simulink model "EulerPIDTunning"  (Simulink 7.6)
settings: Solver=ode3  StartTime=0.0  StopTime=2  FixedStep=Ts  RelTol=1e-3
InitFcn:
  | eval('Config');
  | eval('RobotCtlCfg');
values from neighbouring files (symbols this model uses):
  a2 = 0    [Config.m]    (also in CtrPlatformCfg.m)
  a3 = 0    [Config.m]    (also in CtrPlatformCfg.m)
  a4 = 0    [Config.m]    (also in CtrPlatformCfg.m)
  a5 = 90    [Config.m]    (also in CtrPlatformCfg.m)
  a6 = 0    [Config.m]    (also in CtrPlatformCfg.m)
  freq = tvel/radius    (= 1)    [Config.m]    (also in CtrPlatformCfg.m)
  Gravity = 9.8    [Config.m]    (also in CtrPlatformCfg.m)
  in1 = [5.2954 -0.2565 -0.6366;-0.2565 4.7000 0.2830;-0.6366 0.2829 5.8635]    [Config.m]    (also in CtrPlatformCfg.m; DynEulerTest.m; EfDynCAD.m = [0.54  -0.01 0.23)
  in2 = [5.8840 0.0072 0.0135;0.0072 6.0178 -0.1907;0.0135 -0.1907 0.3374]    [Config.m]    (also in CtrPlatformCfg.m; DynEulerTest.m; EfDynCAD.m = (R_x*R_z)*in2*(R_x*R_z)')
  in3 = [1.8201 -0.2274 -0.3112;-0.2274 2.2537 -0.1441;-0.3112 -0.1441 1.9485]    [Config.m]    (also in CtrPlatformCfg.m; DynEulerTest.m; EfDynCAD.m = (R_x*R_z)*in3*(R_x*R_z)')
  in4 = [0.0607 -0.0922 0;-0.0922 1.4493 0;0 0 1.4620]    [Config.m]    (also in CtrPlatformCfg.m; DynEulerTest.m = [0.0607 -0.0922 0;-0.0922 1.4493 0;0 0,1.4620]; EfDynCAD.m = (R_y*Rz)*in4*(R_y*Rz)')
  in5 = [0.0191 0.0032 0;0.0032 0.0228 0;0 0 0.0291]    [Config.m]    (also in CtrPlatformCfg.m; DynEulerTest.m; EfDynCAD.m = (R_x*R_y)*in5*(R_x*R_y)')
  in6 = [0.0012 0 0;0 0.0007 0;0 0 0.0007]    [Config.m]    (also in CtrPlatformCfg.m; DynEulerTest.m; EfDynCAD.m = (R_y*Rz)*in6*(R_y*Rz)')
  init_Endx = gd_init(1,4)    [Config.m]    (also in CtrPlatformCfg.m)
  init_Endy = gd_init(2,4)    [Config.m]    (also in CtrPlatformCfg.m)
  init_Endz = gd_init(3,4)    [Config.m]    (also in CtrPlatformCfg.m)
  init_Rot = gd_init(1:3,1:3)    [Config.m]    (also in CtrPlatformCfg.m)
  L = [l1 l2 l3 l4 l5 l6 l7 l8 l9]    [Config.m]    (also in CtrPlatformCfg.m)
  ma1 = 170.31    [Config.m]    (also in CtrPlatformCfg.m; DynEulerTest.m; EfDynCAD.m = 77.75)
  ma2 = 63.74    [Config.m]    (also in CtrPlatformCfg.m; DynEulerTest.m; EfDynCAD.m = 32.31)
  ma3 = 98.98    [Config.m]    (also in CtrPlatformCfg.m; DynEulerTest.m; EfDynCAD.m = 18.61)
  ma4 = 24.46    [Config.m]    (also in CtrPlatformCfg.m; DynEulerTest.m; EfDynCAD.m = 15.65)
  ma5 = 5.24    [Config.m]    (also in CtrPlatformCfg.m; DynEulerTest.m; EfDynCAD.m = 3.32)
  ma6 = 0.6    [Config.m]    (also in CtrPlatformCfg.m; DynEulerTest.m; EfDynCAD.m)
  Rad2Line = Gear*EncRes/(2*pi)    [Config.m]    (also in CtrPlatformCfg.m)
  Ts = 1/FrHz    (= 0.00025)    [Config.m]    (also in CtrPlatformCfg.m)
  tvel = 120    [Config.m]    (also in CtrPlatformCfg.m)
undefined symbols (not defined in the file or in its folder): a1, DiscIntNeverNeededParam, PRBSGain, PRBSOffset, PRBSTimeLength, PulseFrq, PulseGain, RobotAxis, SineFrq, SineGain, V2T
libraries: simulink x55, mblibv1 x35, powerlib_extras x7
(part 1 of 3)
settings Model: Creator=DAI Dan  LastModifiedBy=DAI Dan
settings SimMechanicsCC: VisOnUpdateDiagram=on

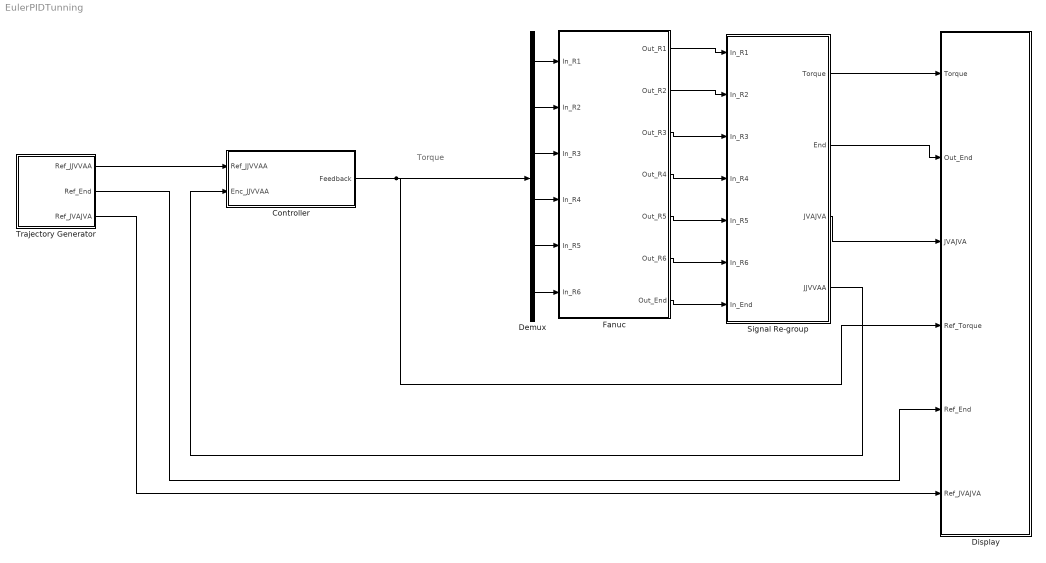
== system EulerPIDTunning ==
  note: Torque
  Controller : Subsystem
  Demux : Demux  Outputs=6
  Display : Subsystem
  Fanuc : Subsystem
  Signal Re-group : Subsystem
  Trajectory Generator : Subsystem
  wires:
  Fanuc/1(Out_R1) -> Signal Re-group/1(In_R1)
  Fanuc/2(Out_R2) -> Signal Re-group/2(In_R2)
  Fanuc/3(Out_R3) -> Signal Re-group/3(In_R3)
  Fanuc/4(Out_R4) -> Signal Re-group/4(In_R4)
  Fanuc/5(Out_R5) -> Signal Re-group/5(In_R5)
  Fanuc/6(Out_R6) -> Signal Re-group/6(In_R6)
  Fanuc/7(Out_End) -> Signal Re-group/7(In_End)
  Signal Re-group/4(JJVVAA) -> Controller/2(Enc_JJVVAA)
  Demux/1 -> Fanuc/1(In_R1)
  Demux/2 -> Fanuc/2(In_R2)
  Demux/3 -> Fanuc/3(In_R3)
  Demux/4 -> Fanuc/4(In_R4)
  Demux/5 -> Fanuc/5(In_R5)
  Demux/6 -> Fanuc/6(In_R6)
  Signal Re-group/1(Torque) -> Display/1(Torque)
  Signal Re-group/2(End) -> Display/2(Out_End)
  Signal Re-group/3(JVAJVA) -> Display/3(JVAJVA)
  Trajectory Generator/1(Ref_JJVVAA) -> Controller/1(Ref_JJVVAA)
  Trajectory Generator/2(Ref_End) -> Display/5(Ref_End)
  Trajectory Generator/3(Ref_JVAJVA) -> Display/6(Ref_JVAJVA)
  Controller/1(Feedback) -> Display/4(Ref_Torque), Demux/1

== system EulerPIDTunning/Controller ==
  note: Note:
      | AugPD controller
      |  Input: rad
      | Output: N*m
      | PID Controller
      | Input: rad-->lines
      | Output: N*m-->Current/Volt
  Ref_JJVVAA : Inport
  Enc_JJVVAA : Inport  Port=2
  PID Controller : Subsystem
  Terminator : Terminator
  Feedback : Outport
  wires:
  Ref_JJVVAA/1 -> PID Controller/1(Ref)
  Enc_JJVVAA/1 -> PID Controller/2(Enc)
  PID Controller/1(Feedback) -> Feedback/1
  PID Controller/2(ErrorFlag) -> Terminator/1

== system EulerPIDTunning/Display ==
  Torque : Inport
  Out_End : Inport  Port=2
  JVAJVA : Inport  Port=3
  Ref_Torque : Inport  Port=4
  Ref_End : Inport  Port=5
  Ref_JVAJVA : Inport  Port=6
  EndTrjDisplay : Subsystem
  JntVelAccDisplay : Subsystem
  TorqueDisplay : Subsystem
  wires:
  Torque/1 -> TorqueDisplay/1(Torque)
  Ref_Torque/1 -> TorqueDisplay/2(Ref_Torque)
  JVAJVA/1 -> JntVelAccDisplay/1(JointVelAcc)
  Ref_JVAJVA/1 -> JntVelAccDisplay/2(Ref_JntVelAcc)
  Out_End/1 -> EndTrjDisplay/1(End)
  Ref_End/1 -> EndTrjDisplay/2(RefEnd)

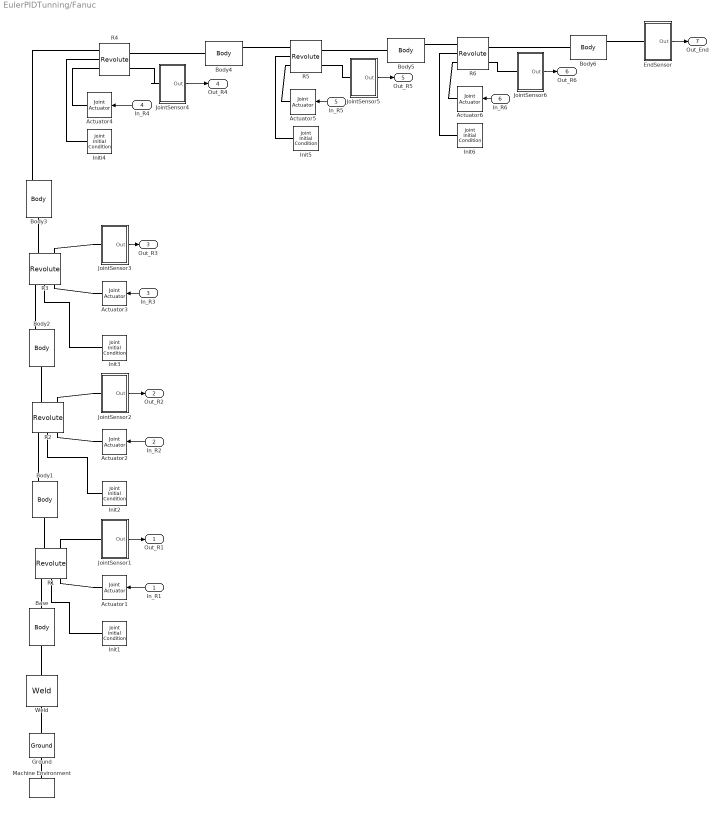
== system EulerPIDTunning/Fanuc ==
  In_R1 : Inport
  In_R2 : Inport  Port=2
  In_R3 : Inport  Port=3
  In_R4 : Inport  Port=4
  In_R5 : Inport  Port=5
  In_R6 : Inport  Port=6
  " EndSensor" : Subsystem
  Actuator{1..6} (6 alike) : mblibv1/Sensors &  Actuators/Joint Actuator  DialogController=MECH.DynMechDlgSource  SystemSampleTime=-1  UpdateFromCAD=off  PhysicalDomain=Mechanical  PortType=blob  ActuationStyle=Force  AngleUnits=rad  ArcVelocityUnits=rad/s  ArcAccelerationUnits=rad/s^2  CoordPositionUnits=m  VelocityUnits=m/s  AccelerationUnits=m/s^2  ForceUnits=N  TorqueUnits=N*m  ActiveIO=on  Width=1  DialogClass=MechanicalActuatorBlock  Primitive=R1  ReferenceFrame=Absolute (World)
  Base : mblibv1/Bodies/Body  DialogController=MECH.DynMechDlgSource  PhysicalDomain=mechanical  SubClassName=Unknown  LeftPortType=workingframe  RightPortType=workingframe  LConnTagsString=CS1  RConnTagsString=CS2  UpdateFromCAD=on  DialogClass=MechanicalBodyBlock  Mass=133.95  MassUnits=kg  InertiaUnits=kg*m^2  Inertia=[3.0977 0.0155 -0.0939;0.0155 3.3580 0.0061;-0.0939 0.0061 5.1969]  Shape=Cylinder  ShapeDims=[1 1]  ShapeUnits=m  ShapeUse=false  Density=1  DensityUnits=kg/m^3  DensityUse=false  GraphicsMode=GFXFILE  GraphicsFileName=M-710iC50 M-710iC70 - M-710iC50 M-710iC70 base-1.STL  BodyColorSelMode=COLORPALETTE  BodyColor=[0.25098 0.25098 0.25098]  AttachedToCS=CS1  CG=Right$CG$[-0.0437 -0.0026 0.1059]$WORLD$WORLD$m$[1 0 0;0 1 0;0 0 1]$3x3 Transform$rad$WORLD$false$none  WorkingFrames=Left$CS1$[0 0 0]$WORLD$WORLD$m$[1 0 0;0 1 0;0 0 1]$3x3 Transform$rad$WORLD$true$none#Right$CS2$[0 0 0.266]$WORLD$WORLD$m$[1 0 0;0 1 0;0 0 1]$3x3 Transform$rad$WORLD$true$none  CGPos=[-0.0437 -0.0026 0.1059]  CGRot=[1 0 0;0 1 0;0 0 1]  CS0Pos=[]  CS0Rot=[]  CS1Pos=[0 0 0]  CS1Rot=[1 0 0;0 1 0;0 0 1]  CS2Pos=[0 0 0.266]  CS2Rot=[1 0 0;0 1 0;0 0 1]  CS3Pos=[]  CS3Rot=[]  CS4Pos=[]  CS4Rot=[]  CS5Pos=[]  CS5Rot=[]  CS6Pos=[]  CS6Rot=[]  CS7Pos=[]  CS7Rot=[]  CS8Pos=[]  CS8Rot=[]  CS9Pos=[]  CS9Rot=[]  CS10Pos=[]  CS10Rot=[]  CS11Pos=[]  CS11Rot=[]  CS12Pos=[]  CS12Rot=[]  CS13Pos=[]  CS13Rot=[]  CS14Pos=[]  CS14Rot=[]  CS15Pos=[]  CS15Rot=[]  CS16Pos=[]  CS16Rot=[]  CS17Pos=[]  CS17Rot=[]  CS18Pos=[]  CS18Rot=[]  CS19Pos=[]  CS19Rot=[]  CS20Pos=[]  CS20Rot=[]
  Body1 : mblibv1/Bodies/Body  DialogController=MECH.DynMechDlgSource  PhysicalDomain=mechanical  SubClassName=Unknown  LeftPortType=workingframe  RightPortType=workingframe  LConnTagsString=CS2  RConnTagsString=CS3|CS4  UpdateFromCAD=on  DialogClass=MechanicalBodyBlock  Mass=ma1  MassUnits=kg  InertiaUnits=kg*m^2  Inertia=in1  Shape=Cylinder  ShapeDims=[1 1]  ShapeUnits=m  ShapeUse=false  Density=1  DensityUnits=kg/m^3  DensityUse=false  GraphicsMode=GFXFILE  GraphicsFileName=M-710iC50 M-710iC70 - M-710iC50 M-710iC70 axis1-1.STL  BodyColorSelMode=COLORPALETTE  BodyColor=[0.86667 0.86667 0.8902]  AttachedToCS=CS1  CG=Right$CG$cen1$WORLD$WORLD$m$[1 0 0;0 1 0;0 0 1]$3x3 Transform$rad$WORLD$false$none  WorkingFrames=Right$CS1$cen1_1$WORLD$WORLD$m$[1 0 0;0 1 0;0 0 1]$3x3 Transform$rad$WORLD$false$none#Left$CS2$cen1_2$WORLD$WORLD$m$[1 0 0;0 1 0;0 0 1]$3x3 Transform$rad$WORLD$true$none#Right$CS3$cen1_3$WORLD$WORLD$m$[1 0 0;0 1 0;0 0 1]$3x3 Transform$rad$WORLD$true$none#Right$CS4$cen1_4$WORLD$WORLD$m$[1 0 0;0 1 0;0 0 1]$3x3 Transform$rad$WORLD$true$none  CGPos=cen1  CGRot=[1 0 0;0 1 0;0 0 1]  CS0Pos=[]  CS0Rot=[]  CS1Pos=cen1_1  CS1Rot=[1 0 0;0 1 0;0 0 1]  CS2Pos=cen1_2  CS2Rot=[1 0 0;0 1 0;0 0 1]  CS3Pos=cen1_3  CS3Rot=[1 0 0;0 1 0;0 0 1]  CS4Pos=cen1_4  CS4Rot=[1 0 0;0 1 0;0 0 1]  CS5Pos=[]  CS5Rot=[]  CS6Pos=[]  CS6Rot=[]  CS7Pos=[]  CS7Rot=[]  CS8Pos=[]  CS8Rot=[]  CS9Pos=[]  CS9Rot=[]  CS10Pos=[]  CS10Rot=[]  CS11Pos=[]  CS11Rot=[]  CS12Pos=[]  CS12Rot=[]  CS13Pos=[]  CS13Rot=[]  CS14Pos=[]  CS14Rot=[]  CS15Pos=[]  CS15Rot=[]  CS16Pos=[]  CS16Rot=[]  CS17Pos=[]  CS17Rot=[]  CS18Pos=[]  CS18Rot=[]  CS19Pos=[]  CS19Rot=[]  CS20Pos=[]  CS20Rot=[]
  Body2 : mblibv1/Bodies/Body  DialogController=MECH.DynMechDlgSource  PhysicalDomain=mechanical  SubClassName=Unknown  LeftPortType=workingframe  RightPortType=workingframe  LConnTagsString=CS2  RConnTagsString=CS3|CS4  UpdateFromCAD=on  DialogClass=MechanicalBodyBlock  Mass=ma2  MassUnits=kg  InertiaUnits=kg*m^2  Inertia=in2  Shape=Cylinder  ShapeDims=[1 1]  ShapeUnits=m  ShapeUse=false  Density=1  DensityUnits=kg/m^3  DensityUse=false  GraphicsMode=GFXFILE  GraphicsFileName=M-710iC50 M-710iC70 - M-710iC50 M-710iC70 axis2-1.STL  BodyColorSelMode=COLORPALETTE  BodyColor=[1 1 0]  AttachedToCS=CS1  CG=Right$CG$cen2$WORLD$WORLD$m$[1 0 0;0 1 0;0 0 1]$3x3 Transform$rad$WORLD$false$none  WorkingFrames=Right$CS1$cen2_1$WORLD$WORLD$m$[1 0 0;0 1 0;0 0 1]$3x3 Transform$rad$WORLD$false$none#Left$CS2$cen2_2$WORLD$WORLD$m$[1 0 0;0 1 0;0 0 1]$3x3 Transform$rad$WORLD$true$none#Right$CS3$cen2_3$WORLD$WORLD$m$[1 0 0;0 1 0;0 0 1]$3x3 Transform$rad$WORLD$true$none#Right$CS4$cen2_4$WORLD$WORLD$m$[1 0 0;0 1 0;0 0 1]$3x3 Transform$rad$WORLD$true$none  CGPos=cen2  CGRot=[1 0 0;0 1 0;0 0 1]  CS0Pos=[]  CS0Rot=[]  CS1Pos=cen2_1  CS1Rot=[1 0 0;0 1 0;0 0 1]  CS2Pos=cen2_2  CS2Rot=[1 0 0;0 1 0;0 0 1]  CS3Pos=cen2_3  CS3Rot=[1 0 0;0 1 0;0 0 1]  CS4Pos=cen2_4  CS4Rot=[1 0 0;0 1 0;0 0 1]  CS5Pos=[]  CS5Rot=[]  CS6Pos=[]  CS6Rot=[]  CS7Pos=[]  CS7Rot=[]  CS8Pos=[]  CS8Rot=[]  CS9Pos=[]  CS9Rot=[]  CS10Pos=[]  CS10Rot=[]  CS11Pos=[]  CS11Rot=[]  CS12Pos=[]  CS12Rot=[]  CS13Pos=[]  CS13Rot=[]  CS14Pos=[]  CS14Rot=[]  CS15Pos=[]  CS15Rot=[]  CS16Pos=[]  CS16Rot=[]  CS17Pos=[]  CS17Rot=[]  CS18Pos=[]  CS18Rot=[]  CS19Pos=[]  CS19Rot=[]  CS20Pos=[]  CS20Rot=[]
  Body3 : mblibv1/Bodies/Body  DialogController=MECH.DynMechDlgSource  PhysicalDomain=mechanical  SubClassName=Unknown  LeftPortType=workingframe  RightPortType=workingframe  LConnTagsString=CS2  RConnTagsString=CS3|CS4  UpdateFromCAD=on  DialogClass=MechanicalBodyBlock  Mass=ma3  MassUnits=kg  InertiaUnits=kg*m^2  Inertia=in3  Shape=Cylinder  ShapeDims=[1 1]  ShapeUnits=m  ShapeUse=false  Density=1  DensityUnits=kg/m^3  DensityUse=false  GraphicsMode=GFXFILE  GraphicsFileName=M-710iC50 M-710iC70 - M-710iC50 M-710iC70 axis3-1.STL  BodyColorSelMode=COLORPALETTE  BodyColor=[1 1 0]  AttachedToCS=CS1  CG=Right$CG$cen3$WORLD$WORLD$m$[1 0 0;0 1 0;0 0 1]$3x3 Transform$rad$WORLD$false$none  WorkingFrames=Right$CS1$cen3_1$WORLD$WORLD$m$[1 0 0;0 1 0;0 0 1]$3x3 Transform$rad$WORLD$false$none#Left$CS2$cen3_2$WORLD$WORLD$m$[1 0 0;0 1 0;0 0 1]$3x3 Transform$rad$WORLD$true$none#Right$CS3$cen3_3$WORLD$WORLD$m$[1 0 0;0 1 0;0 0 1]$3x3 Transform$rad$WORLD$true$none#Right$CS4$cen3_4$WORLD$WORLD$m$[1 0 0;0 1 0;0 0 1]$3x3 Transform$rad$WORLD$true$none  CGPos=cen3  CGRot=[1 0 0;0 1 0;0 0 1]  CS0Pos=[]  CS0Rot=[]  CS1Pos=cen3_1  CS1Rot=[1 0 0;0 1 0;0 0 1]  CS2Pos=cen3_2  CS2Rot=[1 0 0;0 1 0;0 0 1]  CS3Pos=cen3_3  CS3Rot=[1 0 0;0 1 0;0 0 1]  CS4Pos=cen3_4  CS4Rot=[1 0 0;0 1 0;0 0 1]  CS5Pos=[]  CS5Rot=[]  CS6Pos=[]  CS6Rot=[]  CS7Pos=[]  CS7Rot=[]  CS8Pos=[]  CS8Rot=[]  CS9Pos=[]  CS9Rot=[]  CS10Pos=[]  CS10Rot=[]  CS11Pos=[]  CS11Rot=[]  CS12Pos=[]  CS12Rot=[]  CS13Pos=[]  CS13Rot=[]  CS14Pos=[]  CS14Rot=[]  CS15Pos=[]  CS15Rot=[]  CS16Pos=[]  CS16Rot=[]  CS17Pos=[]  CS17Rot=[]  CS18Pos=[]  CS18Rot=[]  CS19Pos=[]  CS19Rot=[]  CS20Pos=[]  CS20Rot=[]
  Body4 : mblibv1/Bodies/Body  DialogController=MECH.DynMechDlgSource  PhysicalDomain=mechanical  SubClassName=Unknown  LeftPortType=workingframe  RightPortType=workingframe  LConnTagsString=CS2  RConnTagsString=CS3|CS4  UpdateFromCAD=on  DialogClass=MechanicalBodyBlock  Mass=ma4  MassUnits=kg  InertiaUnits=kg*m^2  Inertia=in4  Shape=Cylinder  ShapeDims=[1 1]  ShapeUnits=m  ShapeUse=false  Density=1  DensityUnits=kg/m^3  DensityUse=false  GraphicsMode=GFXFILE  GraphicsFileName=M-710iC50 M-710iC70 - M-710iC50 M-710iC70 axis4-1.STL  BodyColorSelMode=COLORPALETTE  BodyColor=[1 1 0]  AttachedToCS=CS1  CG=Right$CG$cen4$WORLD$WORLD$m$[1 0 0;0 0 1;0 -1 0]$3x3 Transform$rad$WORLD$false$none  WorkingFrames=Right$CS1$cen4_1$WORLD$WORLD$m$[1 0 0;0 0 1;0 -1 0]$3x3 Transform$rad$WORLD$false$none#Left$CS2$cen4_2$WORLD$WORLD$m$[1 0 0;0 1 0;0 0 1]$3x3 Transform$rad$WORLD$true$none#Right$CS3$cen4_3$WORLD$WORLD$m$[1 0 0;0 1 0;0 0 1]$3x3 Transform$rad$WORLD$true$none#Right$CS4$cen4_4$WORLD$WORLD$m$[1 0 0;0 1 0;0 0 1]$3x3 Transform$rad$WORLD$true$none  CGPos=cen4  CGRot=[1 0 0;0 0 1;0 -1 0]  CS0Pos=[]  CS0Rot=[]  CS1Pos=cen4_1  CS1Rot=[1 0 0;0 0 1;0 -1 0]  CS2Pos=cen4_2  CS2Rot=[1 0 0;0 1 0;0 0 1]  CS3Pos=cen4_3  CS3Rot=[1 0 0;0 1 0;0 0 1]  CS4Pos=cen4_4  CS4Rot=[1 0 0;0 1 0;0 0 1]  CS5Pos=[]  CS5Rot=[]  CS6Pos=[]  CS6Rot=[]  CS7Pos=[]  CS7Rot=[]  CS8Pos=[]  CS8Rot=[]  CS9Pos=[]  CS9Rot=[]  CS10Pos=[]  CS10Rot=[]  CS11Pos=[]  CS11Rot=[]  CS12Pos=[]  CS12Rot=[]  CS13Pos=[]  CS13Rot=[]  CS14Pos=[]  CS14Rot=[]  CS15Pos=[]  CS15Rot=[]  CS16Pos=[]  CS16Rot=[]  CS17Pos=[]  CS17Rot=[]  CS18Pos=[]  CS18Rot=[]  CS19Pos=[]  CS19Rot=[]  CS20Pos=[]  CS20Rot=[]
  Body5 : mblibv1/Bodies/Body  DialogController=MECH.DynMechDlgSource  PhysicalDomain=mechanical  SubClassName=Unknown  LeftPortType=workingframe  RightPortType=workingframe  LConnTagsString=CS2  RConnTagsString=CS3|CS4  UpdateFromCAD=on  DialogClass=MechanicalBodyBlock  Mass=ma5  MassUnits=kg  InertiaUnits=kg*m^2  Inertia=in5  Shape=Cylinder  ShapeDims=[1 1]  ShapeUnits=m  ShapeUse=false  Density=1  DensityUnits=kg/m^3  DensityUse=false  GraphicsMode=GFXFILE  GraphicsFileName=M-710iC50 M-710iC70 - M-710iC50 M-710iC70 axis5-1.STL  BodyColorSelMode=COLORPALETTE  BodyColor=[1 1 0]  AttachedToCS=CS1  CG=Right$CG$cen5$WORLD$WORLD$m$[1 0 0;0 1 0;0 0 1]$3x3 Transform$rad$WORLD$false$none  WorkingFrames=Right$CS1$cen5_1$WORLD$WORLD$m$[1 0 0;0 1 0;0 0 1]$3x3 Transform$rad$WORLD$false$none#Left$CS2$cen5_2$WORLD$WORLD$m$[1 0 0;0 1 0;0 0 1]$3x3 Transform$rad$WORLD$true$none#Right$CS3$cen5_3$WORLD$WORLD$m$[1 0 0;0 1 0;0 0 1]$3x3 Transform$rad$WORLD$true$none#Right$CS4$cen5_4$WORLD$WORLD$m$[1 0 0;0 1 0;0 0 1]$3x3 Transform$rad$WORLD$true$none  CGPos=cen5  CGRot=[1 0 0;0 1 0;0 0 1]  CS0Pos=[]  CS0Rot=[]  CS1Pos=cen5_1  CS1Rot=[1 0 0;0 1 0;0 0 1]  CS2Pos=cen5_2  CS2Rot=[1 0 0;0 1 0;0 0 1]  CS3Pos=cen5_3  CS3Rot=[1 0 0;0 1 0;0 0 1]  CS4Pos=cen5_4  CS4Rot=[1 0 0;0 1 0;0 0 1]  CS5Pos=[]  CS5Rot=[]  CS6Pos=[]  CS6Rot=[]  CS7Pos=[]  CS7Rot=[]  CS8Pos=[]  CS8Rot=[]  CS9Pos=[]  CS9Rot=[]  CS10Pos=[]  CS10Rot=[]  CS11Pos=[]  CS11Rot=[]  CS12Pos=[]  CS12Rot=[]  CS13Pos=[]  CS13Rot=[]  CS14Pos=[]  CS14Rot=[]  CS15Pos=[]  CS15Rot=[]  CS16Pos=[]  CS16Rot=[]  CS17Pos=[]  CS17Rot=[]  CS18Pos=[]  CS18Rot=[]  CS19Pos=[]  CS19Rot=[]  CS20Pos=[]  CS20Rot=[]
  Body6 : mblibv1/Bodies/Body  DialogController=MECH.DynMechDlgSource  PhysicalDomain=mechanical  SubClassName=Unknown  LeftPortType=workingframe  RightPortType=workingframe  LConnTagsString=CS2  RConnTagsString=CS3|CS4  UpdateFromCAD=on  DialogClass=MechanicalBodyBlock  Mass=ma6  MassUnits=kg  InertiaUnits=kg*m^2  Inertia=in6  Shape=Cylinder  ShapeDims=[1 1]  ShapeUnits=m  ShapeUse=false  Density=1  DensityUnits=kg/m^3  DensityUse=false  GraphicsMode=GFXFILE  GraphicsFileName=M-710iC50 M-710iC70 - M-710iC50 M-710iC70 axis6-1.STL  BodyColorSelMode=COLORPALETTE  BodyColor=[0.75294 0.75294 0.75294]  AttachedToCS=CS1  CG=Right$CG$cen6$WORLD$WORLD$m$[1 0 0;0 1 0;0 0 1]$3x3 Transform$rad$WORLD$false$none  WorkingFrames=Right$CS1$cen6_1$WORLD$WORLD$m$[0 0 1;0 -1 0;1 0 0]$3x3 Transform$rad$WORLD$false$none#Left$CS2$cen6_2$WORLD$WORLD$m$[1 0 0;0 1 0;0 0 1]$3x3 Transform$rad$WORLD$true$none#Right$CS3$cen6_3$WORLD$WORLD$m$[1 0 0;0 1 0;0 0 1]$3x3 Transform$rad$WORLD$true$none#Right$CS4$cen6_4$WORLD$WORLD$m$[1 0 0;0 1 0;0 0 1]$3x3 Transform$rad$WORLD$true$none  CGPos=cen6  CGRot=[1 0 0;0 1 0;0 0 1]  CS0Pos=[]  CS0Rot=[]  CS1Pos=cen6_1  CS1Rot=[0 0 1;0 -1 0;1 0 0]  CS2Pos=cen6_2  CS2Rot=[1 0 0;0 1 0;0 0 1]  CS3Pos=cen6_3  CS3Rot=[1 0 0;0 1 0;0 0 1]  CS4Pos=cen6_4  CS4Rot=[1 0 0;0 1 0;0 0 1]  CS5Pos=[]  CS5Rot=[]  CS6Pos=[]  CS6Rot=[]  CS7Pos=[]  CS7Rot=[]  CS8Pos=[]  CS8Rot=[]  CS9Pos=[]  CS9Rot=[]  CS10Pos=[]  CS10Rot=[]  CS11Pos=[]  CS11Rot=[]  CS12Pos=[]  CS12Rot=[]  CS13Pos=[]  CS13Rot=[]  CS14Pos=[]  CS14Rot=[]  CS15Pos=[]  CS15Rot=[]  CS16Pos=[]  CS16Rot=[]  CS17Pos=[]  CS17Rot=[]  CS18Pos=[]  CS18Rot=[]  CS19Pos=[]  CS19Rot=[]  CS20Pos=[]  CS20Rot=[]
  Ground : mblibv1/Bodies/Ground  DialogController=MECH.DynMechDlgSource  SystemSampleTime=-1  UpdateFromCAD=on  LeftPortType=env  RightPortType=workingframe  PhysicalDomain=Mechanical  DialogClass=GroundBlock  CoordPosition=[0 0 0]  CoordPositionUnits=m  StateVectorMgrId=2  MachineId=[3 0]  ShowEnvPort=on
      link override _mech_engine/ToBlock2: GotoTag=sim_mech_tag8d75a0291950a803
  Init1 : mblibv1/Sensors &  Actuators/Joint Initial Condition  DialogController=MECH.DynMechDlgSource  SystemSampleTime=-1  UpdateFromCAD=off  LeftPortType=blob  RightPortType=blob  PhysicalDomain=mechanical  DialogClass=InitialConditionBlock  InitialConditions=P1$false$0$m$deg$0$m/s$deg/s#P2$false$0$m$deg$0$m/s$deg/s#P3$false$0$m$deg$0$m/s$deg/s#R1$true$a1$m$deg$0$m/s$deg/s#R2$false$0$m$deg$0$m/s$deg/s#R3$false$0$m$deg$0$m/s$deg/s#S$false$0$m$deg$0$m/s$deg/s  P1PIC=0  P1VIC=0  P2PIC=0  P2VIC=0  P3PIC=0  P3VIC=0  R1PIC=a1  R1VIC=0  R2PIC=0  R2VIC=0  R3PIC=0  R3VIC=0  SPIC=0  SVIC=0
  Init2 : mblibv1/Sensors &  Actuators/Joint Initial Condition  DialogController=MECH.DynMechDlgSource  SystemSampleTime=-1  UpdateFromCAD=off  LeftPortType=blob  RightPortType=blob  PhysicalDomain=mechanical  DialogClass=InitialConditionBlock  InitialConditions=P1$false$0$m$deg$0$m/s$deg/s#P2$false$0$m$deg$0$m/s$deg/s#P3$false$0$m$deg$0$m/s$deg/s#R1$true$a2$m$deg$0$m/s$deg/s#R2$false$0$m$deg$0$m/s$deg/s#R3$false$0$m$deg$0$m/s$deg/s#S$false$0$m$deg$0$m/s$deg/s  P1PIC=0  P1VIC=0  P2PIC=0  P2VIC=0  P3PIC=0  P3VIC=0  R1PIC=a2  R1VIC=0  R2PIC=0  R2VIC=0  R3PIC=0  R3VIC=0  SPIC=0  SVIC=0
  Init3 : mblibv1/Sensors &  Actuators/Joint Initial Condition  DialogController=MECH.DynMechDlgSource  SystemSampleTime=-1  UpdateFromCAD=off  LeftPortType=blob  RightPortType=blob  PhysicalDomain=mechanical  DialogClass=InitialConditionBlock  InitialConditions=P1$false$0$m$deg$0$m/s$deg/s#P2$false$0$m$deg$0$m/s$deg/s#P3$false$0$m$deg$0$m/s$deg/s#R1$true$a3$m$deg$0$m/s$deg/s#R2$false$0$m$deg$0$m/s$deg/s#R3$false$0$m$deg$0$m/s$deg/s#S$false$0$m$deg$0$m/s$deg/s  P1PIC=0  P1VIC=0  P2PIC=0  P2VIC=0  P3PIC=0  P3VIC=0  R1PIC=a3  R1VIC=0  R2PIC=0  R2VIC=0  R3PIC=0  R3VIC=0  SPIC=0  SVIC=0
  Init5 : mblibv1/Sensors &  Actuators/Joint Initial Condition  DialogController=MECH.DynMechDlgSource  SystemSampleTime=-1  UpdateFromCAD=off  LeftPortType=blob  RightPortType=blob  PhysicalDomain=mechanical  DialogClass=InitialConditionBlock  InitialConditions=P1$false$0$m$deg$0$m/s$deg/s#P2$false$0$m$deg$0$m/s$deg/s#P3$false$0$m$deg$0$m/s$deg/s#R1$true$a5$m$deg$0$m/s$deg/s#R2$false$0$m$deg$0$m/s$deg/s#R3$false$0$m$deg$0$m/s$deg/s#S$false$0$m$deg$0$m/s$deg/s  P1PIC=0  P1VIC=0  P2PIC=0  P2VIC=0  P3PIC=0  P3VIC=0  R1PIC=a5  R1VIC=0  R2PIC=0  R2VIC=0  R3PIC=0  R3VIC=0  SPIC=0  SVIC=0
  Init6 : mblibv1/Sensors &  Actuators/Joint Initial Condition  DialogController=MECH.DynMechDlgSource  SystemSampleTime=-1  UpdateFromCAD=off  LeftPortType=blob  RightPortType=blob  PhysicalDomain=mechanical  DialogClass=InitialConditionBlock  InitialConditions=P1$false$0$m$deg$0$m/s$deg/s#P2$false$0$m$deg$0$m/s$deg/s#P3$false$0$m$deg$0$m/s$deg/s#R1$true$a6$m$deg$0$m/s$deg/s#R2$false$0$m$deg$0$m/s$deg/s#R3$false$0$m$deg$0$m/s$deg/s#S$false$0$m$deg$0$m/s$deg/s  P1PIC=0  P1VIC=0  P2PIC=0  P2VIC=0  P3PIC=0  P3VIC=0  R1PIC=a6  R1VIC=0  R2PIC=0  R2VIC=0  R3PIC=0  R3VIC=0  SPIC=0  SVIC=0
  Initi4 : mblibv1/Sensors &  Actuators/Joint Initial Condition  DialogController=MECH.DynMechDlgSource  SystemSampleTime=-1  UpdateFromCAD=off  LeftPortType=blob  RightPortType=blob  PhysicalDomain=mechanical  DialogClass=InitialConditionBlock  InitialConditions=P1$false$0$m$deg$0$m/s$deg/s#P2$false$0$m$deg$0$m/s$deg/s#P3$false$0$m$deg$0$m/s$deg/s#R1$true$a4$m$deg$0$m/s$deg/s#R2$false$0$m$deg$0$m/s$deg/s#R3$false$0$m$deg$0$m/s$deg/s#S$false$0$m$deg$0$m/s$deg/s  P1PIC=0  P1VIC=0  P2PIC=0  P2VIC=0  P3PIC=0  P3VIC=0  R1PIC=a4  R1VIC=0  R2PIC=0  R2VIC=0  R3PIC=0  R3VIC=0  SPIC=0  SVIC=0
  JointSensor1 : Subsystem
  JointSensor2 : Subsystem
  JointSensor3 : Subsystem
  JointSensor4 : Subsystem
  JointSensor5 : Subsystem
  JointSensor6 : Subsystem
  Machine Environment : mblibv1/Bodies/Machine Environment  DialogController=MECH.DialogSource  SystemSampleTime=-1  PortType=env  PhysicalDomain=Mechanical  DialogTemplateClass=MECH.MachineEnvironment  SyncWhenCopied=off  Gravity=[0 0 Gravity]  GravityUnits=m/s^2  GravityAsSignal=off  Dimensionality=Auto-detect  AnalysisType=Forward dynamics  LinearAssemblyTolerance=1e-3  LinearAssemblyToleranceUnits=m  AngularAssemblyTolerance=1e-3  AngularAssemblyToleranceUnits=rad  ConstraintSolverType=Stabilizing  ConstraintRelTolerance=1e-4  ConstraintAbsTolerance=1e-4  UseRobustSingularityHandling=off  RedundancyAnalysisToleranceType=Automatically select tolerance  RedundancyAnalysisTolerance=1e-14  StatePerturbationType=Fixed  PerturbationSize=1e-5  VisualizeMachine=on  BodyVisualizationType=Use model default body geometries  BodyColorSelMode=Use model default  DefaultBodyColor=[1 0 0]
  R1 : mblibv1/Joints/Revolute  DialogController=MECH.DynMechDlgSource  PhysicalDomain=mechanical  SubClassName=Unknown  LeftPortType=blob  RightPortType=blob  LConnTagsString=__newl0|SA1|SA2  RConnTagsString=__newr0|SA1  UpdateFromCAD=on  NumSAPorts=3  CutJoint=off  MarkAsCut=off  Primitives=prismatic  PrimitiveProps=R1$World$[0,0,1]$revolute  DialogClass=JointBlock  R1Axis=[0,0,1]
  R2 : mblibv1/Joints/Revolute  DialogController=MECH.DynMechDlgSource  PhysicalDomain=mechanical  SubClassName=Unknown  LeftPortType=blob  RightPortType=blob  LConnTagsString=__newl0|SA1|SA2  RConnTagsString=__newr0|SA1  UpdateFromCAD=on  NumSAPorts=3  CutJoint=off  MarkAsCut=off  Primitives=prismatic  PrimitiveProps=R1$World$[0,1,0]$revolute  DialogClass=JointBlock  R1Axis=[0,1,0]
  R3 : mblibv1/Joints/Revolute  DialogController=MECH.DynMechDlgSource  PhysicalDomain=mechanical  SubClassName=Unknown  LeftPortType=blob  RightPortType=blob  LConnTagsString=__newl0|SA1|SA2  RConnTagsString=__newr0|SA1  UpdateFromCAD=on  NumSAPorts=3  CutJoint=off  MarkAsCut=off  Primitives=prismatic  PrimitiveProps=R1$World$[0,1,0]$revolute  DialogClass=JointBlock  R1Axis=[0,1,0]
  R4 : mblibv1/Joints/Revolute  DialogController=MECH.DynMechDlgSource  PhysicalDomain=mechanical  SubClassName=Unknown  LeftPortType=blob  RightPortType=blob  LConnTagsString=__newl0|SA1|SA2  RConnTagsString=__newr0|SA1  UpdateFromCAD=on  NumSAPorts=3  CutJoint=off  MarkAsCut=off  Primitives=prismatic  PrimitiveProps=R1$World$[1,0,0]$revolute  DialogClass=JointBlock  R1Axis=[1,0,0]
  R5 : mblibv1/Joints/Revolute  DialogController=MECH.DynMechDlgSource  PhysicalDomain=mechanical  SubClassName=Unknown  LeftPortType=blob  RightPortType=blob  LConnTagsString=__newl0|SA1|SA2  RConnTagsString=__newr0|SA1  UpdateFromCAD=on  NumSAPorts=3  CutJoint=off  MarkAsCut=off  Primitives=prismatic  PrimitiveProps=R1$World$[0,1,0]$revolute  DialogClass=JointBlock  R1Axis=[0,1,0]
  R6 : mblibv1/Joints/Revolute  DialogController=MECH.DynMechDlgSource  PhysicalDomain=mechanical  SubClassName=Unknown  LeftPortType=blob  RightPortType=blob  LConnTagsString=__newl0|SA1|SA2  RConnTagsString=__newr0|SA1  UpdateFromCAD=on  NumSAPorts=3  CutJoint=off  MarkAsCut=off  Primitives=prismatic  PrimitiveProps=R1$World$[1,0,0]$revolute  DialogClass=JointBlock  R1Axis=[1,0,0]
  Weld : mblibv1/Joints/Weld  DialogController=MECH.DynMechDlgSource  PhysicalDomain=mechanical  SubClassName=Unknown  LeftPortType=blob  RightPortType=blob  LConnTagsString=__newl0  RConnTagsString=__newr0  UpdateFromCAD=on  NumSAPorts=0  CutJoint=off  MarkAsCut=off  Primitives=weld  PrimitiveProps=W$WORLD$[0.57735,0.57735,0.57735]$weld  DialogClass=JointBlock  WAxis=[0.57735,0.57735,0.57735]
  Out_R1 : Outport
  Out_R2 : Outport  Port=2
  Out_R3 : Outport  Port=3
  Out_R4 : Outport  Port=4
  Out_R5 : Outport  Port=5
  Out_R6 : Outport  Port=6
  Out_End : Outport  Port=7
  wires:
  In_R1/1 -> Actuator1/1
  In_R2/1 -> Actuator2/1
  JointSensor2/1(Out) -> Out_R2/1
  In_R3/1 -> Actuator3/1
  JointSensor3/1(Out) -> Out_R3/1
  JointSensor4/1(Out) -> Out_R4/1
  In_R4/1 -> Actuator4/1
  JointSensor5/1(Out) -> Out_R5/1
  In_R5/1 -> Actuator5/1
  In_R6/1 -> Actuator6/1
  " EndSensor"/1(Out) -> Out_End/1
  JointSensor1/1(Out) -> Out_R1/1
  JointSensor6/1(Out) -> Out_R6/1
  connections:
  " EndSensor"/LConn1 -- Body6/RConn1
  JointSensor6/LConn1 -- R6/RConn2
  Actuator6/RConn1 -- R6/LConn3
  Weld/LConn1 -- Ground/RConn1
  Actuator3/RConn1 -- R3/LConn3
  Init3/RConn1 -- R3/LConn2
  JointSensor3/LConn1 -- R3/RConn2
  Machine Environment/RConn1 -- Ground/LConn1
  R5/LConn1 -- Body4/RConn1
  R1/LConn1 -- Base/RConn1
  R6/RConn1 -- Body6/LConn1
  R5/RConn1 -- Body5/LConn1
  Body5/RConn1 -- R6/LConn1
  Body2/RConn1 -- R3/LConn1
  R2/RConn1 -- Body2/LConn1
  R2/LConn1 -- Body1/RConn1
  Weld/RConn1 -- Base/LConn1
  Actuator2/RConn1 -- R2/LConn3
  Init6/RConn1 -- R6/LConn2
  Body1/LConn1 -- R1/RConn1
  JointSensor2/LConn1 -- R2/RConn2
  Init2/RConn1 -- R2/LConn2
  R1/RConn2 -- JointSensor1/LConn1
  Actuator1/RConn1 -- R1/LConn3
  R1/LConn2 -- Init1/RConn1
  JointSensor5/LConn1 -- R5/RConn2
  R3/RConn1 -- Body3/LConn1
  Actuator5/RConn1 -- R5/LConn3
  Init5/RConn1 -- R5/LConn2
  R4/RConn1 -- Body4/LConn1
  R4/LConn1 -- Body3/RConn1
  Actuator4/RConn1 -- R4/LConn3
  Initi4/RConn1 -- R4/LConn2
  JointSensor4/LConn1 -- R4/RConn2

== system EulerPIDTunning/Signal Re-group ==
  In_R1 : Inport
  In_R2 : Inport  Port=2
  In_R3 : Inport  Port=3
  In_R4 : Inport  Port=4
  In_R5 : Inport  Port=5
  In_R6 : Inport  Port=6
  In_End : Inport  Port=7
  Deg2Rad : Gain  Gain=pi/180
  Re-group : Subsystem
  Re-group JntVelAcc : Subsystem
  Re-group_R1 : Subsystem
  Re-group_R2 : Subsystem
  Re-group_R3 : Subsystem
  Re-group_R4 : Subsystem
  Re-group_R5 : Subsystem
  Re-group_R6 : Subsystem
  Torque : Outport
  End : Outport  Port=2
  JVAJVA : Outport  Port=3
  JJVVAA : Outport  Port=4
  wires:
  In_R1/1 -> Re-group_R1/1(In_R1)
  In_R2/1 -> Re-group_R2/1(In_R2)
  In_R3/1 -> Re-group_R3/1(In_R3)
  In_R4/1 -> Re-group_R4/1(In_R4)
  In_R5/1 -> Re-group_R5/1(In_R5)
  In_R6/1 -> Re-group_R6/1(In_R6)
  Re-group/1(JntVelAcc) -> JVAJVA/1, Re-group JntVelAcc/1(JntVelAcc)
  Re-group/2(Torque) -> Torque/1
  In_End/1 -> End/1
  Re-group JntVelAcc/1(ReJntVelAcc) -> Deg2Rad/1
  Deg2Rad/1 -> JJVVAA/1
  Re-group_R1/1(JntVelAcc_R1) -> Re-group/1(JntVelAcc_R1)
  Re-group_R1/2(Torque_R1) -> Re-group/2(Torque_R1)
  Re-group_R2/1(JntVelAcc_R2) -> Re-group/3(JntVelAcc_R2)
  Re-group_R2/2(Torque_R2) -> Re-group/4(Torque_R2)
  Re-group_R3/1(JntVelAcc_R3) -> Re-group/5(JntVelAcc_R3)
  Re-group_R3/2(Torque_R3) -> Re-group/6(Torque_R3)
  Re-group_R4/1(JntVelAcc_R4) -> Re-group/7(JntVelAcc_R4)
  Re-group_R4/2(Torque_R4) -> Re-group/8(Torque_R4)
  Re-group_R5/1(JntVelAcc_R5) -> Re-group/9(JntVelAcc_R5)
  Re-group_R5/2(Torque_R5) -> Re-group/10(Torque_R5)
  Re-group_R6/1(JntVelAcc_R6) -> Re-group/11(JntVelAcc_R6)
  Re-group_R6/2(Torque_R6) -> Re-group/12(Torque_R6)

== system EulerPIDTunning/Trajectory Generator ==
  Circle in Descartes Space : Subsystem
  End Switch : MultiPortSwitch  zeroidx=off
  JJVVAA Switch : MultiPortSwitch  zeroidx=off
  JVA Switch : MultiPortSwitch  zeroidx=off
  Line in Joint Space : Subsystem
  Still : Subsystem
  Switch : Constant  SampleTime=Ts
  Ref_JJVVAA : Outport
  Ref_End : Outport  Port=2
  Ref_JVAJVA : Outport  Port=3
  wires:
  Switch/1 -> JJVVAA Switch/1, End Switch/1, JVA Switch/1
  Circle in Descartes Space/1(Ref_JJVVAA) -> JJVVAA Switch/2
  Still/1(Ref_JJVVAA) -> JJVVAA Switch/3
  Line in Joint Space/1(Ref_JJVVAA) -> JJVVAA Switch/4
  Circle in Descartes Space/2(RefEnd) -> End Switch/2
  Still/2(RefEnd) -> End Switch/3
  Line in Joint Space/2(RefEnd) -> End Switch/4
  Circle in Descartes Space/3(Ref_JVAJVA) -> JVA Switch/2
  Still/3(Ref_JVAJVA) -> JVA Switch/3
  Line in Joint Space/3(Ref_JVAJVA) -> JVA Switch/4
  JJVVAA Switch/1 -> Ref_JJVVAA/1
  End Switch/1 -> Ref_End/1
  JVA Switch/1 -> Ref_JVAJVA/1

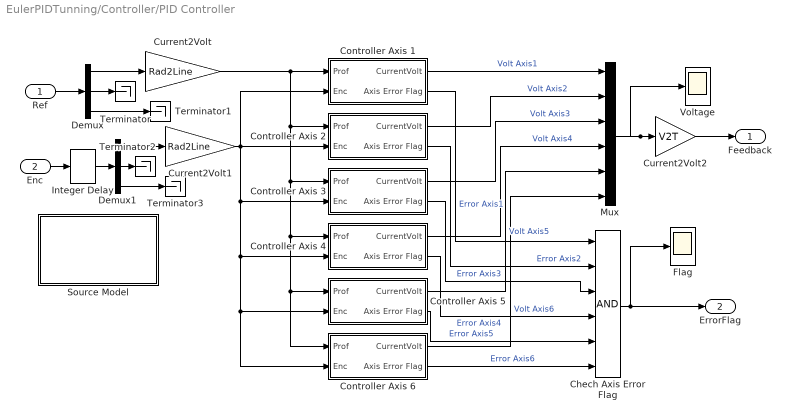
== system EulerPIDTunning/Controller/PID Controller ==
  Ref : Inport
  Enc : Inport  Port=2
  Chech Axis Error Flag : Logic  Inputs=6  AllPortsSameDT=off  OutDataTypeStr=boolean
  Controller Axis 1 : Subsystem  mask{RobotAxis=RobotAxis(1), Ts=Ts}
      mask prompts: RobotAxis "Robot Axis Controller Parameter"; Ts "Sample Time"
      mask init:
      | %% Source and Control Loop Selection
      | iPosCtl=RobotAxis.PosSourceSelect;
      | iVelCtl=RobotAxis.VelSourceSelect;
      | iCurrentCtl=RobotAxis.CurrentSourceSelect;
      | AxisNO=RobotAxis.AxisNO;
      | 
      | %% Controller Parameter
      | PLKp=RobotAxis.PLKp; % Kp for position loop
      | PLLimit=RobotAxis.PLLimit; 
      | 
      | VLKp = RobotAxis.VLKp; % Kp for velocity loop
      | VLKi = RobotAxis.VLKi;
      | VLLimit = RobotAxis.VLLimit;
      | 
      | Current2Volt=RobotAxis.Current2Volt;
      | 
      | %% Protection
      | VelErrorCheckLimit=RobotAxis.VelErrorCheckLimit;
  Controller Axis 2 : Subsystem  mask{RobotAxis=RobotAxis(2), Ts=Ts}
      mask prompts: RobotAxis "Robot Axis Controller Parameter"; Ts "Sample Time"
      mask init: same as EulerPIDTunning/Controller/PID Controller/Controller Axis 1
  Controller Axis 3 : Subsystem  mask{RobotAxis=RobotAxis(3), Ts=Ts}
      mask prompts: RobotAxis "Robot Axis Controller Parameter"; Ts "Sample Time"
      mask init: same as EulerPIDTunning/Controller/PID Controller/Controller Axis 1
  Controller Axis 4 : Subsystem  mask{RobotAxis=RobotAxis(4), Ts=Ts}
      mask prompts: RobotAxis "Robot Axis Controller Parameter"; Ts "Sample Time"
      mask init: same as EulerPIDTunning/Controller/PID Controller/Controller Axis 1
  Controller Axis 5 : Subsystem  mask{RobotAxis=RobotAxis(5), Ts=Ts}
      mask prompts: RobotAxis "Robot Axis Controller Parameter"; Ts "Sample Time"
      mask init: same as EulerPIDTunning/Controller/PID Controller/Controller Axis 1
  Controller Axis 6 : Subsystem  mask{RobotAxis=RobotAxis(6), Ts=Ts}
      mask prompts: RobotAxis "Robot Axis Controller Parameter"; Ts "Sample Time"
      mask init: same as EulerPIDTunning/Controller/PID Controller/Controller Axis 1
  Current2Volt : Gain  Gain=Rad2Line  SampleTime=Ts
  Current2Volt1 : Gain  Gain=Rad2Line  SampleTime=Ts
  Current2Volt2 : Gain  Gain=V2T
  Demux : Demux  Outputs=3
  Demux1 : Demux  Outputs=3
  Flag : Scope
      settings: TimeRange=12  YMin=-9  YMax=9
  Integer Delay : simulink/Discrete/Integer Delay  NumDelays=1  vinit=[a1;a2;a3;a4;a5;a6;0;0;0;0;0;0;0;0;0;0;0;0]/180*pi  samptime=Ts
  Mux : Mux  Inputs=6
  Source Model : Subsystem
  Terminator{,1..3} (4 alike) : Terminator
  Voltage : Scope
      settings: TimeRange=12  YMin=-9  YMax=9
  Feedback : Outport
  ErrorFlag : Outport  Port=2
  wires:
  Controller Axis 1/1(CurrentVolt) -> Mux/1  "Volt Axis1"
  Controller Axis 2/1(CurrentVolt) -> Mux/2  "Volt Axis2"
  Controller Axis 3/1(CurrentVolt) -> Mux/3  "Volt Axis3"
  Controller Axis 4/1(CurrentVolt) -> Mux/4  "Volt Axis4"
  Controller Axis 5/1(CurrentVolt) -> Mux/5  "Volt Axis5"
  Controller Axis 6/1(CurrentVolt) -> Mux/6  "Volt Axis6"
  Mux/1 -> Voltage/1, Current2Volt2/1
  Controller Axis 1/2(Axis Error Flag) -> Chech Axis Error Flag/1  "Error Axis1"
  Controller Axis 2/2(Axis Error Flag) -> Chech Axis Error Flag/2  "Error Axis2"
  Controller Axis 3/2(Axis Error Flag) -> Chech Axis Error Flag/3  "Error Axis3"
  Controller Axis 4/2(Axis Error Flag) -> Chech Axis Error Flag/4  "Error Axis4"
  Controller Axis 5/2(Axis Error Flag) -> Chech Axis Error Flag/5  "Error Axis5"
  Controller Axis 6/2(Axis Error Flag) -> Chech Axis Error Flag/6  "Error Axis6"
  Chech Axis Error Flag/1 -> ErrorFlag/1, Flag/1
  Current2Volt/1 -> Controller Axis 6/1(Prof), Controller Axis 5/1(Prof), Controller Axis 4/1(Prof), Controller Axis 3/1(Prof), Controller Axis 2/1(Prof), Controller Axis 1/1(Prof)
  Current2Volt1/1 -> Controller Axis 6/2(Enc), Controller Axis 5/2(Enc), Controller Axis 4/2(Enc), Controller Axis 3/2(Enc), Controller Axis 1/2(Enc), Controller Axis 2/2(Enc)
  Current2Volt2/1 -> Feedback/1
  Ref/1 -> Demux/1
  Demux/1 -> Current2Volt/1
  Demux/2 -> Terminator/1
  Demux/3 -> Terminator1/1
  Demux1/1 -> Current2Volt1/1
  Demux1/2 -> Terminator2/1
  Demux1/3 -> Terminator3/1
  Enc/1 -> Integer Delay/1
  Integer Delay/1 -> Demux1/1

== system EulerPIDTunning/Display/EndTrjDisplay ==
  End : Inport
  RefEnd : Inport  Port=2
  Demux : Demux  Outputs=5
  Demux1 : Demux  Outputs=5
  EndAccDisplay : Subsystem
  EndPosDisplay : Subsystem
  EndVelDisplay : Subsystem
  Mux{,1..3} (4 alike) : Mux  Inputs=2
  wires:
  End/1 -> Demux/1
  Demux/2 -> Mux/1
  Demux/3 -> Mux/2
  Demux/4 -> Mux1/1
  Demux/5 -> Mux1/2
  Demux1/2 -> Mux2/1
  Demux1/3 -> Mux2/2
  Demux1/4 -> Mux3/1
  Demux1/5 -> Mux3/2
  RefEnd/1 -> Demux1/1
  Demux/1 -> EndPosDisplay/1(EndPos)
  Demux1/1 -> EndPosDisplay/2(Ref_EndPos)
  Mux/1 -> EndVelDisplay/1(EndVel)
  Mux2/1 -> EndVelDisplay/2(Ref_EndVel)
  Mux1/1 -> EndAccDisplay/1(EndAcc)
  Mux3/1 -> EndAccDisplay/2(Ref_EndAcc)

== system EulerPIDTunning/Display/JntVelAccDisplay ==
  JointVelAcc : Inport
  Ref_JntVelAcc : Inport  Port=2
  Demux1 : Demux  Outputs=6
  Demux3 : Demux  Outputs=6
  Joint1 : Subsystem
  Joint2 : Subsystem
  Joint3 : Subsystem
  Joint4 : Subsystem
  Joint5 : Subsystem
  Joint6 : Subsystem
  wires:
  Demux1/6 -> Joint6/2(Ref_JVA6)
  Demux3/6 -> Joint6/1(JVA6)
  Demux1/5 -> Joint5/2(Ref_JVA5)
  Demux3/5 -> Joint5/1(JVA5)
  Demux1/4 -> Joint4/2(Ref_JVA4)
  Demux3/4 -> Joint4/1(JVA4)
  Demux1/3 -> Joint3/2(Ref_JVA3)
  Demux3/3 -> Joint3/1(JVA3)
  Demux1/2 -> Joint2/2(Ref_JVA2)
  Demux3/2 -> Joint2/1(JVA2)
  Demux3/1 -> Joint1/1(JVA1)
  Demux1/1 -> Joint1/2(Ref_JVA1)
  Ref_JntVelAcc/1 -> Demux1/1
  JointVelAcc/1 -> Demux3/1

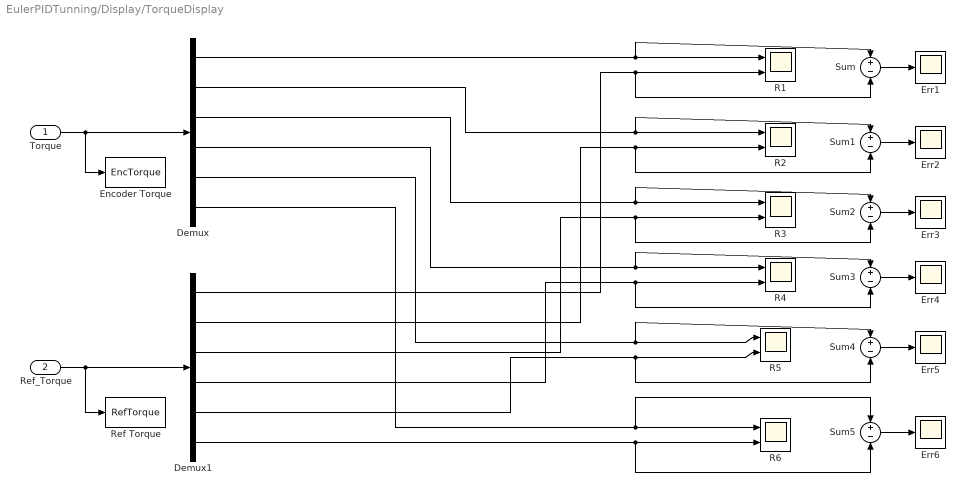
== system EulerPIDTunning/Display/TorqueDisplay ==
  Torque : Inport
  Ref_Torque : Inport  Port=2
  Demux : Demux  Outputs=6
  Demux1 : Demux  Outputs=6
  Encoder Torque : ToWorkspace  VariableName=EncTorque  SampleTime=-1  SaveFormat=Structure
  Err{1..6} (6 alike) : Scope
      Err1 settings: SaveName=ScopeData6
      Err2 settings: SaveName=ScopeData7
      Err3 settings: SaveName=ScopeData8
      Err4 settings: SaveName=ScopeData9
      Err5 settings: TimeRange=3  YMin=-2.5  YMax=1  SaveName=ScopeData10
      Err6 settings: SaveName=ScopeData11
  R{1,3..6} (5 alike) : Scope  NumInputPorts=2
      R1 settings: TimeRange=10  YMin=-2.999999999999999e-017~-1  YMax=4e-017~1
      R3 settings: YMin=-5~-5  YMax=5~5  SaveName=ScopeData2
      R4 settings: YMin=-5~-5  YMax=5~5  SaveName=ScopeData3
      R5 settings: TimeRange=10  YMin=-4.18~4.060000000000001  YMax=-4.04~4.2  SaveName=ScopeData4
      R6 settings: TimeRange=10  YMin=-1.6e-006~-0.003  YMax=4e-007~0.004  SaveName=ScopeData5
  "R2 " : Scope  NumInputPorts=2
      settings: YMin=-5~-5  YMax=5~5
  Ref Torque : ToWorkspace  VariableName=RefTorque  SampleTime=-1  SaveFormat=Structure
  Sum{,1..5} (6 alike) : Sum  Inputs=+|-
  wires:
  Sum/1 -> Err1/1
  Sum1/1 -> Err2/1
  Sum2/1 -> Err3/1
  Sum3/1 -> Err4/1
  Sum4/1 -> Err5/1
  Sum5/1 -> Err6/1
  Torque/1 -> Demux/1, Encoder Torque/1
  Ref_Torque/1 -> Demux1/1, Ref Torque/1
  Demux/1 -> Sum/1, R1/1
  Demux1/1 -> Sum/2, R1/2
  Demux/2 -> "R2 "/1, Sum1/1
  Demux/3 -> R3/1, Sum2/1
  Demux/4 -> Sum3/1, R4/1
  Demux/5 -> R5/1, Sum4/1
  Demux/6 -> R6/1, Sum5/1
  Demux1/2 -> "R2 "/2, Sum1/2
  Demux1/3 -> R3/2, Sum2/2
  Demux1/4 -> Sum3/2, R4/2
  Demux1/5 -> R5/2, Sum4/2
  Demux1/6 -> R6/2, Sum5/2

== system EulerPIDTunning/Fanuc/ EndSensor ==
  Avx : Scope
      settings: TimeRange=3  YMin=-150  YMax=125  SaveName=ScopeData62
  Avy : Scope
      settings: TimeRange=3  YMin=-150  YMax=125  SaveName=ScopeData63
  Avz : Scope
      settings: TimeRange=3  YMin=-150  YMax=125  SaveName=ScopeData64
  Awx : Scope
      settings: TimeRange=3  YMin=-150  YMax=125  SaveName=ScopeData65
  Awy : Scope
      settings: TimeRange=3  YMin=-150  YMax=125  SaveName=ScopeData66
  Awz : Scope
      settings: TimeRange=3  YMin=-150  YMax=125  SaveName=ScopeData67
  "Body Sensor " : mblibv1/Sensors &  Actuators/Body Sensor  DialogController=MECH.DynMechDlgSource  SystemSampleTime=-1  UpdateFromCAD=off  PhysicalDomain=Mechanical  PortType=blob  Muxed=on  Pose=off  Angle=on  AngleUnits=deg  ArcVelocity=on  ArcVelocityUnits=deg/s  ArcAcceleration=on  ArcAccelerationUnits=deg/s^2  CoordPosition=on  CoordPositionUnits=mm  Velocity=on  VelocityUnits=mm/s  Acceleration=on  AccelerationUnits=mm/s^2  Quaternion=on  QuaternionDT=off  QuaternionDDT=off  QuaternionUnits=off  OutputVector=[1]  ActiveIO=on  Width=15  DialogClass=MechanicalSensorBlock  ReferenceFrame=Absolute (World)
  Demux5 : Demux  Outputs=15
  EndX : ToWorkspace  VariableName=EndX  SampleTime=-1  SaveFormat=Structure
  EndY : ToWorkspace  VariableName=EndY  SampleTime=-1  SaveFormat=Structure
  EndZ : ToWorkspace  VariableName=EndZ  SampleTime=-1  SaveFormat=Structure
  Vx : Scope
      settings: TimeRange=3  YMin=-150  YMax=125  SaveName=ScopeData55
  Vy : Scope
      settings: TimeRange=3  YMin=-150  YMax=125  SaveName=ScopeData57
  Vz : Scope
      settings: TimeRange=3  YMin=-150  YMax=125  SaveName=ScopeData58
  X : Scope
      settings: TimeRange=3  YMin=-150  YMax=125  SaveName=ScopeData36
  Y : Scope
      settings: TimeRange=3  YMin=-150  YMax=125  SaveName=ScopeData37
  Z : Scope
      settings: TimeRange=3  YMin=-150  YMax=125  SaveName=ScopeData38
  wx : Scope
      settings: TimeRange=3  YMin=-150  YMax=125  SaveName=ScopeData59
  wy : Scope
      settings: TimeRange=3  YMin=-150  YMax=125  SaveName=ScopeData60
  wz : Scope
      settings: TimeRange=3  YMin=-150  YMax=125  SaveName=ScopeData61
  In : PMIOPort  Port=1  Side=Left
  Out : Outport
  wires:
  "Body Sensor "/1 -> Demux5/1, Out/1
  Demux5/4 -> Vx/1
  Demux5/5 -> Vy/1
  Demux5/6 -> Vz/1
  Demux5/7 -> wx/1
  Demux5/8 -> wy/1
  Demux5/9 -> wz/1
  Demux5/10 -> Avx/1
  Demux5/11 -> Avy/1
  Demux5/12 -> Avz/1
  Demux5/13 -> Awx/1
  Demux5/14 -> Awy/1
  Demux5/15 -> Awz/1
  Demux5/1 -> EndX/1, X/1
  Demux5/2 -> EndY/1, Y/1
  Demux5/3 -> EndZ/1, Z/1
  connections:
  In/RConn1 -- "Body Sensor "/LConn1

== system EulerPIDTunning/Fanuc/JointSensor1 ==
  Angle Acceleration : Scope
      settings: SaveName=ScopeData32
  Angle Velocity : Scope
      settings: SaveName=ScopeData31
  Anlge : Scope
      settings: SaveName=ScopeData30
  Computed Torque : Scope
      settings: SaveName=ScopeData33
  Demux : Demux
  Sensor1 : mblibv1/Sensors &  Actuators/Joint Sensor  DialogController=MECH.DynMechDlgSource  SystemSampleTime=-1  UpdateFromCAD=off  PhysicalDomain=Mechanical  PortType=blob  Muxed=on  Pose=off  Angle=on  AngleUnits=deg  ArcVelocity=on  ArcVelocityUnits=deg/s  ArcAcceleration=on  ArcAccelerationUnits=deg/s^2  CoordPosition=on  CoordPositionUnits=m  Velocity=off  VelocityUnits=m/s  Acceleration=off  AccelerationUnits=m/s^2  Quaternion=on  QuaternionDT=off  QuaternionDDT=off  QuaternionUnits=off  OutputVector=[1]  ActiveIO=on  Width=4  DialogClass=MechanicalSensorBlock  Primitive=R1  Force=off  ForceUnits=N  Torque=on  TorqueUnits=N*m  ReferenceFrame=Absolute (World)  ReactionSensedSide=Follower  ReactionReferenceFrame=Absolute (World)  ReactionForce=off  ReactionForceUnits=N  ReactionMoment=off  ReactionMomentUnits=N*m
  In : PMIOPort  Port=1  Side=Left
  Out : Outport
  wires:
  Demux/4 -> Computed Torque/1
  Demux/3 -> Angle Acceleration/1
  Demux/1 -> Anlge/1
  Demux/2 -> Angle Velocity/1
  Sensor1/1 -> Out/1, Demux/1
  connections:
  In/RConn1 -- Sensor1/LConn1

== system EulerPIDTunning/Fanuc/JointSensor2 ==
  Angle Acceleration : Scope
      settings: SaveName=ScopeData32
  Angle Velocity : Scope
      settings: SaveName=ScopeData31
  Anlge : Scope
      settings: SaveName=ScopeData30
  Computed Torque : Scope
      settings: SaveName=ScopeData33
  Demux : Demux
  Sensor1 : mblibv1/Sensors &  Actuators/Joint Sensor  DialogController=MECH.DynMechDlgSource  SystemSampleTime=-1  UpdateFromCAD=off  PhysicalDomain=Mechanical  PortType=blob  Muxed=on  Pose=off  Angle=on  AngleUnits=deg  ArcVelocity=on  ArcVelocityUnits=deg/s  ArcAcceleration=on  ArcAccelerationUnits=deg/s^2  CoordPosition=on  CoordPositionUnits=m  Velocity=off  VelocityUnits=m/s  Acceleration=off  AccelerationUnits=m/s^2  Quaternion=on  QuaternionDT=off  QuaternionDDT=off  QuaternionUnits=off  OutputVector=[1]  ActiveIO=on  Width=4  DialogClass=MechanicalSensorBlock  Primitive=R1  Force=off  ForceUnits=N  Torque=on  TorqueUnits=N*m  ReferenceFrame=Absolute (World)  ReactionSensedSide=Follower  ReactionReferenceFrame=Absolute (World)  ReactionForce=off  ReactionForceUnits=N  ReactionMoment=off  ReactionMomentUnits=N*m
  In : PMIOPort  Port=1  Side=Left
  Out : Outport
  wires:
  Demux/4 -> Computed Torque/1
  Demux/3 -> Angle Acceleration/1
  Demux/1 -> Anlge/1
  Demux/2 -> Angle Velocity/1
  Sensor1/1 -> Out/1, Demux/1
  connections:
  In/RConn1 -- Sensor1/LConn1

== system EulerPIDTunning/Fanuc/JointSensor3 ==
  Angle Acceleration : Scope
      settings: SaveName=ScopeData32
  Angle Velocity : Scope
      settings: SaveName=ScopeData31
  Anlge : Scope
      settings: SaveName=ScopeData30
  Computed Torque : Scope
      settings: SaveName=ScopeData33
  Demux : Demux
  Sensor1 : mblibv1/Sensors &  Actuators/Joint Sensor  DialogController=MECH.DynMechDlgSource  SystemSampleTime=-1  UpdateFromCAD=off  PhysicalDomain=Mechanical  PortType=blob  Muxed=on  Pose=off  Angle=on  AngleUnits=deg  ArcVelocity=on  ArcVelocityUnits=deg/s  ArcAcceleration=on  ArcAccelerationUnits=deg/s^2  CoordPosition=on  CoordPositionUnits=m  Velocity=off  VelocityUnits=m/s  Acceleration=off  AccelerationUnits=m/s^2  Quaternion=on  QuaternionDT=off  QuaternionDDT=off  QuaternionUnits=off  OutputVector=[1]  ActiveIO=on  Width=4  DialogClass=MechanicalSensorBlock  Primitive=R1  Force=off  ForceUnits=N  Torque=on  TorqueUnits=N*m  ReferenceFrame=Absolute (World)  ReactionSensedSide=Follower  ReactionReferenceFrame=Absolute (World)  ReactionForce=off  ReactionForceUnits=N  ReactionMoment=off  ReactionMomentUnits=N*m
  In : PMIOPort  Port=1  Side=Left
  Out : Outport
  wires:
  Demux/4 -> Computed Torque/1
  Demux/3 -> Angle Acceleration/1
  Demux/1 -> Anlge/1
  Demux/2 -> Angle Velocity/1
  Sensor1/1 -> Out/1, Demux/1
  connections:
  In/RConn1 -- Sensor1/LConn1

== system EulerPIDTunning/Fanuc/JointSensor4 ==
  Angle Acceleration : Scope
      settings: SaveName=ScopeData32
  Angle Velocity : Scope
      settings: SaveName=ScopeData31
  Anlge : Scope
      settings: SaveName=ScopeData30
  Computed Torque : Scope
      settings: SaveName=ScopeData33
  Demux : Demux
  Sensor1 : mblibv1/Sensors &  Actuators/Joint Sensor  DialogController=MECH.DynMechDlgSource  SystemSampleTime=-1  UpdateFromCAD=off  PhysicalDomain=Mechanical  PortType=blob  Muxed=on  Pose=off  Angle=on  AngleUnits=deg  ArcVelocity=on  ArcVelocityUnits=deg/s  ArcAcceleration=on  ArcAccelerationUnits=deg/s^2  CoordPosition=on  CoordPositionUnits=m  Velocity=off  VelocityUnits=m/s  Acceleration=off  AccelerationUnits=m/s^2  Quaternion=on  QuaternionDT=off  QuaternionDDT=off  QuaternionUnits=off  OutputVector=[1]  ActiveIO=on  Width=4  DialogClass=MechanicalSensorBlock  Primitive=R1  Force=off  ForceUnits=N  Torque=on  TorqueUnits=N*m  ReferenceFrame=Absolute (World)  ReactionSensedSide=Follower  ReactionReferenceFrame=Absolute (World)  ReactionForce=off  ReactionForceUnits=N  ReactionMoment=off  ReactionMomentUnits=N*m
  In : PMIOPort  Port=1  Side=Left
  Out : Outport
  wires:
  Demux/4 -> Computed Torque/1
  Demux/3 -> Angle Acceleration/1
  Demux/1 -> Anlge/1
  Demux/2 -> Angle Velocity/1
  Sensor1/1 -> Out/1, Demux/1
  connections:
  In/RConn1 -- Sensor1/LConn1

== system EulerPIDTunning/Fanuc/JointSensor5 ==
  Angle Acceleration : Scope
      settings: SaveName=ScopeData32
  Angle Velocity : Scope
      settings: SaveName=ScopeData31
  Anlge : Scope
      settings: SaveName=ScopeData30
  Computed Torque : Scope
      settings: SaveName=ScopeData33
  Demux : Demux
  Sensor1 : mblibv1/Sensors &  Actuators/Joint Sensor  DialogController=MECH.DynMechDlgSource  SystemSampleTime=-1  UpdateFromCAD=off  PhysicalDomain=Mechanical  PortType=blob  Muxed=on  Pose=off  Angle=on  AngleUnits=deg  ArcVelocity=on  ArcVelocityUnits=deg/s  ArcAcceleration=on  ArcAccelerationUnits=deg/s^2  CoordPosition=on  CoordPositionUnits=m  Velocity=off  VelocityUnits=m/s  Acceleration=off  AccelerationUnits=m/s^2  Quaternion=on  QuaternionDT=off  QuaternionDDT=off  QuaternionUnits=off  OutputVector=[1]  ActiveIO=on  Width=4  DialogClass=MechanicalSensorBlock  Primitive=R1  Force=off  ForceUnits=N  Torque=on  TorqueUnits=N*m  ReferenceFrame=Absolute (World)  ReactionSensedSide=Follower  ReactionReferenceFrame=Absolute (World)  ReactionForce=off  ReactionForceUnits=N  ReactionMoment=off  ReactionMomentUnits=N*m
  In : PMIOPort  Port=1  Side=Left
  Out : Outport
  wires:
  Demux/4 -> Computed Torque/1
  Demux/3 -> Angle Acceleration/1
  Demux/1 -> Anlge/1
  Demux/2 -> Angle Velocity/1
  Sensor1/1 -> Out/1, Demux/1
  connections:
  In/RConn1 -- Sensor1/LConn1

== system EulerPIDTunning/Fanuc/JointSensor6 ==
  Angle Acceleration : Scope
      settings: SaveName=ScopeData32
  Angle Velocity : Scope
      settings: SaveName=ScopeData31
  Anlge : Scope
      settings: SaveName=ScopeData30
  Computed Torque : Scope
      settings: SaveName=ScopeData33
  Demux : Demux
  Sensor1 : mblibv1/Sensors &  Actuators/Joint Sensor  DialogController=MECH.DynMechDlgSource  SystemSampleTime=-1  UpdateFromCAD=off  PhysicalDomain=Mechanical  PortType=blob  Muxed=on  Pose=off  Angle=on  AngleUnits=deg  ArcVelocity=on  ArcVelocityUnits=deg/s  ArcAcceleration=on  ArcAccelerationUnits=deg/s^2  CoordPosition=on  CoordPositionUnits=m  Velocity=off  VelocityUnits=m/s  Acceleration=off  AccelerationUnits=m/s^2  Quaternion=on  QuaternionDT=off  QuaternionDDT=off  QuaternionUnits=off  OutputVector=[1]  ActiveIO=on  Width=4  DialogClass=MechanicalSensorBlock  Primitive=R1  Force=off  ForceUnits=N  Torque=on  TorqueUnits=N*m  ReferenceFrame=Absolute (World)  ReactionSensedSide=Follower  ReactionReferenceFrame=Absolute (World)  ReactionForce=off  ReactionForceUnits=N  ReactionMoment=off  ReactionMomentUnits=N*m
  In : PMIOPort  Port=1  Side=Left
  Out : Outport
  wires:
  Demux/4 -> Computed Torque/1
  Demux/3 -> Angle Acceleration/1
  Demux/1 -> Anlge/1
  Demux/2 -> Angle Velocity/1
  Sensor1/1 -> Out/1, Demux/1
  connections:
  In/RConn1 -- Sensor1/LConn1

== system EulerPIDTunning/Signal Re-group/Re-group ==
  JntVelAcc_R1 : Inport
  Torque_R1 : Inport  Port=2
  JntVelAcc_R2 : Inport  Port=3
  Torque_R2 : Inport  Port=4
  JntVelAcc_R3 : Inport  Port=5
  Torque_R3 : Inport  Port=6
  JntVelAcc_R4 : Inport  Port=7
  Torque_R4 : Inport  Port=8
  JntVelAcc_R5 : Inport  Port=9
  Torque_R5 : Inport  Port=10
  JntVelAcc_R6 : Inport  Port=11
  Torque_R6 : Inport  Port=12
  Mux : Mux  Inputs=6
  Mux1 : Mux  Inputs=6
  JntVelAcc : Outport
  Torque : Outport  Port=2
  wires:
  JntVelAcc_R1/1 -> Mux/1
  JntVelAcc_R2/1 -> Mux/2
  JntVelAcc_R3/1 -> Mux/3
  JntVelAcc_R4/1 -> Mux/4
  JntVelAcc_R5/1 -> Mux/5
  JntVelAcc_R6/1 -> Mux/6
  Torque_R1/1 -> Mux1/1
  Torque_R2/1 -> Mux1/2
  Torque_R3/1 -> Mux1/3
  Torque_R4/1 -> Mux1/4
  Torque_R5/1 -> Mux1/5
  Torque_R6/1 -> Mux1/6
  Mux/1 -> JntVelAcc/1
  Mux1/1 -> Torque/1

== system EulerPIDTunning/Signal Re-group/Re-group JntVelAcc ==
  JntVelAcc : Inport
  Demux2 : Demux  Outputs=18
  Mux : Mux  Inputs=6
  Mux1 : Mux  Inputs=6
  Mux2 : Mux  Inputs=6
  Mux3 : Mux  Inputs=3
  ReJntVelAcc : Outport
  wires:
  JntVelAcc/1 -> Demux2/1
  Demux2/1 -> Mux/1
  Demux2/2 -> Mux1/1
  Demux2/3 -> Mux2/1
  Demux2/4 -> Mux/2
  Demux2/5 -> Mux1/2
  Demux2/6 -> Mux2/2
  Demux2/7 -> Mux/3
  Demux2/8 -> Mux1/3
  Demux2/9 -> Mux2/3
  Demux2/10 -> Mux/4
  Demux2/11 -> Mux1/4
  Demux2/12 -> Mux2/4
  Demux2/13 -> Mux/5
  Demux2/14 -> Mux1/5
  Demux2/15 -> Mux2/5
  Demux2/16 -> Mux/6
  Demux2/17 -> Mux1/6
  Demux2/18 -> Mux2/6
  Mux/1 -> Mux3/1
  Mux1/1 -> Mux3/2
  Mux2/1 -> Mux3/3
  Mux3/1 -> ReJntVelAcc/1

== system EulerPIDTunning/Signal Re-group/Re-group_R1 ==
  In_R1 : Inport
  Demux2 : Demux
  Mux : Mux  Inputs=3
  JntVelAcc_R1 : Outport
  Torque_R1 : Outport  Port=2
  wires:
  In_R1/1 -> Demux2/1
  Demux2/1 -> Mux/1
  Demux2/2 -> Mux/2
  Demux2/3 -> Mux/3
  Demux2/4 -> Torque_R1/1
  Mux/1 -> JntVelAcc_R1/1
